simulink model "identifikaciaS"  (R2021a)
settings: Solver=FixedStepAuto  StartTime=0.0  StopTime=stopTime  FixedStep=Ts  RelTol=1e-3
values from neighbouring files (symbols this model uses):
  A = [-2.68660932824  -0.00784455027611; 1  0]    [back.mat]
  B = [1 0]    [back.mat]
  C = [-0.198008601998 2.58763495901]    [back.mat]
  D = 0    [back.mat]
  initVal = 4    [srdce.m]    (also in tlak.m = pFilter(tLvzorka))
  stepTime = 150    [srdce.m]    (also in tlak.m = 133)
  xInit = [0 48.3066591618]    [back.mat]    (also in identFitS.m = [0, init/C(2), 0]; results.m = [0, init/C(2)]; srdce.m = [0, init/C(2), 0])
settings Model: Creator=marko  LastModifiedBy=marko

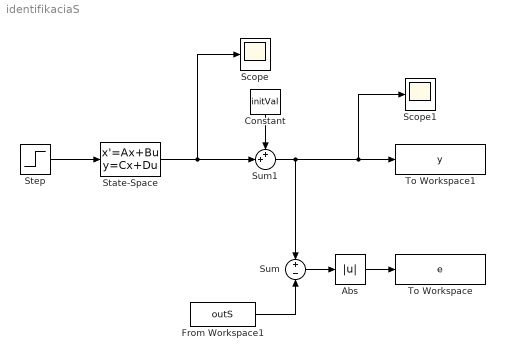
== system identifikaciaS ==
  Abs : Abs
  Constant : Constant  Value=initVal
  From Workspace1 : FromWorkspace  VariableName=outS  Interpolate=off  OutputAfterFinalValue=Holding final value
  Scope : Scope
  Scope1 : Scope
  State-Space : StateSpace  A=A  B=B  C=C  D=D  InitialCondition=xInit
  Step : Step  Time=stepTime  Before=1  After=0  SampleTime=0
  Sum : Sum  Inputs=+|-
  Sum1 : Sum  Inputs=++|
  To Workspace : ToWorkspace  VariableName=e  SampleTime=-1
  To Workspace1 : ToWorkspace  VariableName=y  SaveFormat=Timeseries  SampleTime=-1
  wires:
  From Workspace1/1 -> Sum/2
  Sum/1 -> Abs/1
  Abs/1 -> To Workspace/1
  Step/1 -> State-Space/1
  State-Space/1 -> Scope/1, Sum1/2
  Sum1/1 -> Sum/1, Scope1/1, To Workspace1/1
  Constant/1 -> Sum1/1
